simulink model "MultiPhys_v1"  (R2013a)
settings: Solver=ode45  StartTime=0.0  StopTime=10.0  RelTol=1e-3
libraries: fl_lib x19, elec_lib x5, nesl_utility x3, sh_lib x1
settings Model: Creator=mainster  LastModifiedBy=mainster

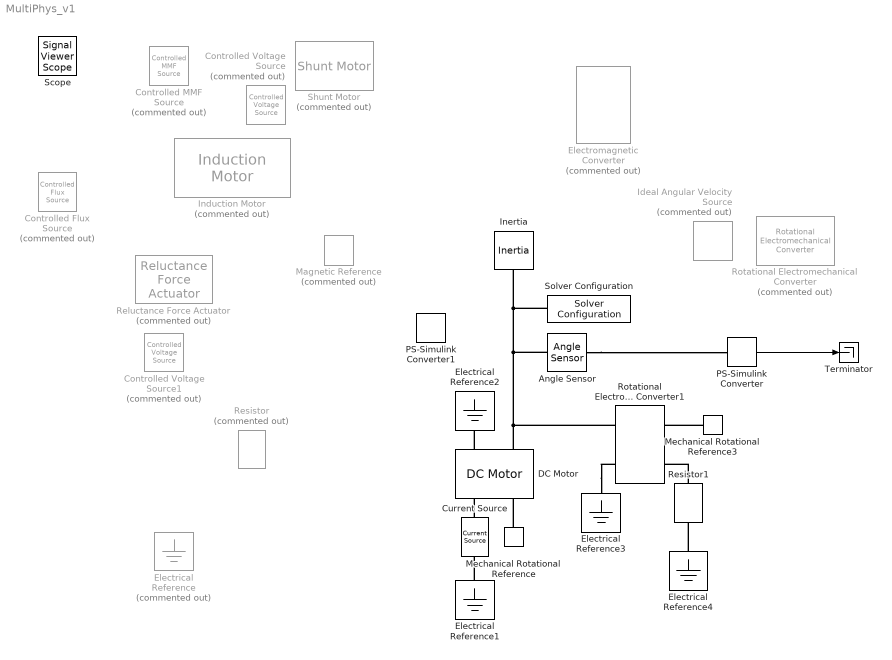
== system MultiPhys_v1 ==
  Angle Sensor : sh_lib/Pumps and Motors/Angle Sensor  phase_angle=0 rad  LocalVarLogging=[]
  Controlled Flux Source : fl_lib/Magnetic/Magnetic Sources/Controlled Flux Source  Commented=on  phi_Log=off  mmf_Log=off  LocalVarNames=|phi|mmf  LocalVarDescs=|phi|mmf  LocalVarLogging=[0 0]
  Controlled MMF Source : fl_lib/Magnetic/Magnetic Sources/Controlled MMF Source  Commented=on  phi_Log=off  mmf_Log=off  LocalVarNames=|phi|mmf  LocalVarDescs=|phi|mmf  LocalVarLogging=[0 0]
  Controlled Voltage Source : fl_lib/Electrical/Electrical Sources/Controlled Voltage Source  Commented=on  i_Log=off  v_Log=off  LocalVarNames=|i|v  LocalVarDescs=|i|v  LocalVarLogging=[0 0]
  Controlled Voltage Source1 : fl_lib/Electrical/Electrical Sources/Controlled Voltage Source  Commented=on  i_Log=off  v_Log=off  LocalVarNames=|i|v  LocalVarDescs=|i|v  LocalVarLogging=[0 0]
  Current Source : elec_lib/Sources/Current Source  dc_current=0 A  ac_current=1 A  ac_shift=0 deg  ac_frequency=100 Hz  noise_mode=0  PSD=0 A^2/Hz  sample_time=0.001 s  repeatability=1  auto_seed=897368659  user_seed=0  LocalVarLogging=[]
  DC Motor : elec_lib/Actuators & Drivers/Rotational Actuators/DC Motor  parameterization=2  Ra=3.9 Ohm  La=160e-6 H  emf_or_torque=1  Kv=7.2e-5 V/rpm  Ki=6.876e-4 N*m/A  T_stall=2.4e-4 N*m  w_max=1.91e+4 rpm  w_rated=1.5e+4 rpm  P_rated=0.08 W  V_rated=1.5 V  J=0.01 g*cm^2  lam_param=1  lam=1e-9 N*m/(rad/s)  i_noload=0 A  V_i_noload=1.5 V  speed0=0 rpm  current_Log=off  voltage_Log=off  power_Log=off  i2r_Log=off  torque_Log=off  speed_Log=off  LocalVarNames=|current|voltage|power|i2r|torque|speed  LocalVarDescs=|Current (A)|Voltage (V)|Power (W)|Electrical losses (W)|Torque (Nm)|Angular speed (rad/s)  LocalVarLogging=[0 0 0 0 0 0]  alpha=0.00393 1/K  Tmeas=25 C  thermal_mass=100 J/K  initial_temperature=25 C
  Electrical Reference : fl_lib/Electrical/Electrical Elements/Electrical Reference  Commented=on  i_Log=off  LocalVarNames=|i  LocalVarDescs=|i  LocalVarLogging=0
  Electrical Reference{1..4} (4 alike) : fl_lib/Electrical/Electrical Elements/Electrical Reference  i_Log=off  LocalVarNames=|i  LocalVarDescs=|i  LocalVarLogging=0
  Electromagnetic Converter : fl_lib/Magnetic/Magnetic Elements/Electromagnetic Converter  Commented=on  Nw=1  i_Log=off  v_Log=off  mmf_Log=off  phi_Log=off  LocalVarNames=|i|v|mmf|phi  LocalVarDescs=|i|v|mmf|phi  LocalVarLogging=[0 0 0 0]
  Ideal Angular Velocity Source : fl_lib/Mechanical/Mechanical Sources/Ideal Angular Velocity Source  Commented=on  w_Log=off  t_Log=off  LocalVarNames=|w|t  LocalVarDescs=|w|t  LocalVarLogging=[0 0]
  Induction Motor : elec_lib/Actuators & Drivers/Rotational Actuators/Induction Motor  Commented=on  param=1  R1=1 Ohm  R2=1 Ohm  L1=0.02 H  L2=0.02 H  Lm=0.5 H  P_rated=825 W  w_mech=3.5e+3 rpm  v_rated=200 V  w_rated=60 Hz  i_rated=2.7 A  paramR1=1  E=95  pf=0.93  R1m=1 Ohm  V=200 V  w=60 Hz  p=1  n=3  paramLoad=1  J=0.001 kg*m^2  lam=1e-4 N*m/(rad/s)  speed0=0 rpm  LocalVarLogging=[]  alpha=[ 0.00393 0.00393 ] 1/K  Tmeas=25 C  thermal_masses=[ 100 100 ] J/K  initial_temperatures=[ 25 25 ] C
  Inertia : fl_lib/Mechanical/Rotational Elements/Inertia  inertia=0.01 kg*m^2  initial_velocity=0 rad/s  t_Log=off  LocalVarNames=|t  LocalVarDescs=|t  LocalVarLogging=0
  Magnetic Reference : fl_lib/Magnetic/Magnetic Elements/Magnetic Reference  Commented=on  phi_Log=off  LocalVarNames=|phi  LocalVarDescs=|phi  LocalVarLogging=0
  Mechanical Rotational Reference : fl_lib/Mechanical/Rotational Elements/Mechanical Rotational Reference  t_Log=off  LocalVarNames=|t  LocalVarDescs=|t  LocalVarLogging=0
  Mechanical Rotational Reference3 : fl_lib/Mechanical/Rotational Elements/Mechanical Rotational Reference  t_Log=off  LocalVarNames=|t  LocalVarDescs=|t  LocalVarLogging=0
  PS-Simulink Converter : nesl_utility/PS-Simulink Converter  PhysicalDomain=network_engine_domain  SubClassName=ps_output  LeftPortType=input  RightPortType=output  PseudoPeriodic=off  Frequencies=[]  Unit=1  AffineConversion=off
  PS-Simulink Converter1 : nesl_utility/PS-Simulink Converter  PhysicalDomain=network_engine_domain  SubClassName=ps_output  LeftPortType=input  RightPortType=output  PseudoPeriodic=off  Frequencies=[]  Unit=1  AffineConversion=off
  Reluctance Force Actuator : fl_lib/Magnetic/Magnetic Elements/Reluctance Force Actuator  Commented=on  x0=2 mm  xmin=1e-4 mm  CSA=0.01 m^2  mur=1  K_contact=1e6 N/m  D_contact=500 N/(m/s)  mmf_Log=off  phi_Log=off  f_Log=off  u_Log=off  x_Log=off  LocalVarNames=|mmf|phi|f|u|x  LocalVarDescs=|mmf|phi|f|u|x  LocalVarLogging=[0 0 0 0 0]
  Resistor : elec_lib/Passive Devices/Resistor  Commented=on  R=1 Ohm  noise_mode=0  Tdevice=25 C  sample_time=0.001 s  repeatability=1  auto_seed=2225016863  user_seed=0  LocalVarLogging=[]
  Resistor1 : fl_lib/Electrical/Electrical Elements/Resistor  R=1 Ohm  i_Log=off  v_Log=off  LocalVarNames=|i|v  LocalVarDescs=|i|v  LocalVarLogging=[0 0]
  Rotational Electromechanical Converter : fl_lib/Electrical/Electrical Elements/Rotational Electromechanical Converter  Commented=on  K=0.1 V/(rad/s)  i_Log=off  v_Log=off  t_Log=off  w_Log=off  LocalVarNames=|i|v|t|w  LocalVarDescs=|i|v|t|w  LocalVarLogging=[0 0 0 0]
  Rotational Electromechanical Converter1 : fl_lib/Electrical/Electrical Elements/Rotational Electromechanical Converter  K=0.1 V/(rad/s)  i_Log=off  v_Log=off  t_Log=off  w_Log=off  LocalVarNames=|i|v|t|w  LocalVarDescs=|i|v|t|w  LocalVarLogging=[0 0 0 0]
  Shunt Motor : elec_lib/Actuators & Drivers/Rotational Actuators/Shunt Motor  Commented=on  parameterization=1  Ra=110 Ohm  Rf=2.5e+3 Ohm  Laf=5.11 s*V/rad/A  w_max=4.6e+3 rpm  w_rated=4e+3 rpm  P_rated=50 W  V_rated=220 V  I_start=2.09 A  La=0.1 H  Lf=0.1 H  J=2e-4 kg*m^2  lam=1e-6 N*m/(rad/s)  speed0=0 rpm  current_Log=off  voltage_Log=off  power_Log=off  i2r_Log=off  torque_Log=off  speed_Log=off  LocalVarNames=|current|voltage|power|i2r|torque|speed  LocalVarDescs=|Current (A)|Voltage (V)|Power (W)|Electrical losses (W)|Torque (Nm)|Angular speed (rad/s)  LocalVarLogging=[0 0 0 0 0 0]  alpha=[ 0.00393 0.00393 ] 1/K  Tmeas=25 C  thermal_masses=[ 100 100 ] J/K  initial_temperatures=[ 25 25 ] C
  Solver Configuration : nesl_utility/Solver Configuration  PhysicalDomain=network_engine_domain  SubClassName=solver  LeftPortType=input  RightPortType=generic  Accelerate=off  Tones=[]  Harmonics=[]  SimulateNoise=off  Profile=off  UseLocalSampling=off  EnableSwitchedLinearOptims=on  FrequencyDomain=off  UseCCode=off  UseNewInitialization=off  DoDC=on  ResidualTolerance=1e-09  UseLocalSolver=on  LocalSolverChoice=NE_BACKWARD_EULER_ADVANCER  LocalSolverSampleTime=0.001  DoFixedCost=on  MaxNonlinIter=3  MaxModeIter=2  LinearAlgebra=Sparse  DelaysMemoryBudget=1024
  Terminator : Terminator
  Scope : SignalViewerScope  IOType=viewer  RefreshTime=0.035000
  wires:
  PS-Simulink Converter/1 -> Terminator/1
  connections:
  Electrical Reference1/LConn1 -- Current Source/LConn1
  Current Source/RConn1 -- DC Motor/RConn1
  DC Motor/LConn1 -- Electrical Reference2/LConn1
  DC Motor/LConn2 -- Rotational Electromechanical Converter1/RConn2 -- Angle Sensor/LConn1 -- Solver Configuration/RConn1 -- Inertia/LConn1
  Mechanical Rotational Reference/LConn1 -- DC Motor/RConn2
  Mechanical Rotational Reference3/LConn1 -- Rotational Electromechanical Converter1/LConn2
  Rotational Electromechanical Converter1/RConn1 -- Electrical Reference3/LConn1
  Resistor1/LConn1 -- Rotational Electromechanical Converter1/LConn1
  Electrical Reference4/LConn1 -- Resistor1/RConn1
  Angle Sensor/RConn1 -- PS-Simulink Converter/LConn1
